simulink model "Linear_Test"  (R2025b)
settings: Solver=ode3  StartTime=0.0  StopTime=10.0  FixedStep=0.005  RelTol=1e-3
undefined symbols (not defined in the file or in its folder): SimPar
settings Model: Creator=bullo  LastModifiedBy=bullo

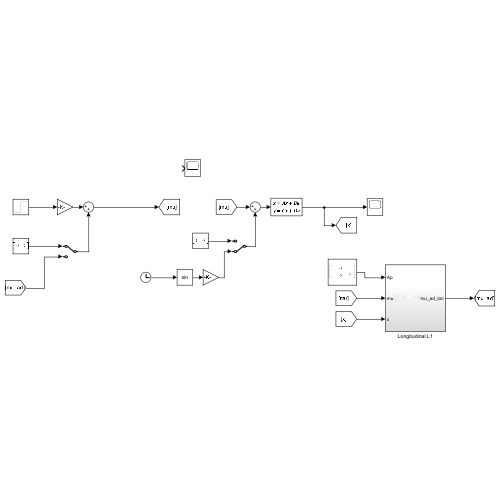
[thumbnail: Simulink's stored preview of the top-level diagram]
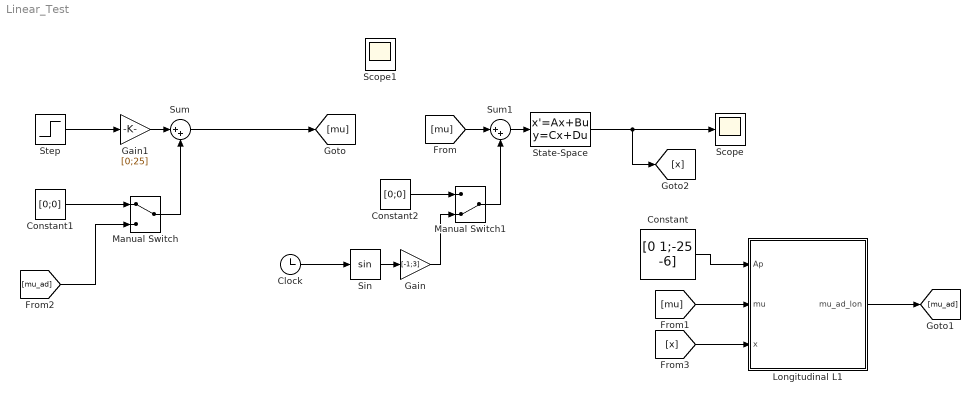
== system Linear_Test ==
  Clock : Clock
  Constant : Constant  Value=[0 1;-25 -6]
  Constant1 : Constant  Value=[0;0]
  Constant2 : Constant  Value=[0;0]
  Gain : Gain  Gain=[-1;3]
  Gain1 : Gain  Gain=[0;25]
  Longitudinal L1 : Subsystem
  Manual Switch : ManualSwitch
  Manual Switch1 : ManualSwitch  CurrentSetting=0
  Scope : Scope
      settings: ActiveDisplayYMinimum=-1.5712970754637268  ActiveDisplayYMaximum=3.9637552838320249
  Scope1 : Scope
      settings: ActiveDisplayYMinimum=-1  ActiveDisplayYMaximum=1
  Sin : Trigonometry
  State-Space : StateSpace  A=[0 1;-25 -6]  B=eye(2)  C=eye(2)  D=zeros(2,2)  InitialCondition=[0;0]
  Step : Step  SampleTime=0
  Sum : Sum  Inputs=|++
  Sum1 : Sum  Inputs=|++
  wires:
  State-Space/1 -> [x], Scope/1
  Constant/1 -> Longitudinal L1/1(Ap)
  [mu] -> Longitudinal L1/2(mu)
  Manual Switch/1 -> Sum/2
  [mu_ad] -> Manual Switch/2
  Longitudinal L1/1(mu_ad_lon) -> [mu_ad]
  [x] -> Longitudinal L1/3(x)
  [mu] -> Sum1/1
  Sum1/1 -> State-Space/1
  Manual Switch1/1 -> Sum1/2
  Constant2/1 -> Manual Switch1/1
  Clock/1 -> Sin/1
  Sin/1 -> Gain/1
  Gain/1 -> Manual Switch1/2
  Constant1/1 -> Manual Switch/1
  Step/1 -> Gain1/1
  Gain1/1 -> Sum/1
  Sum/1 -> [mu]

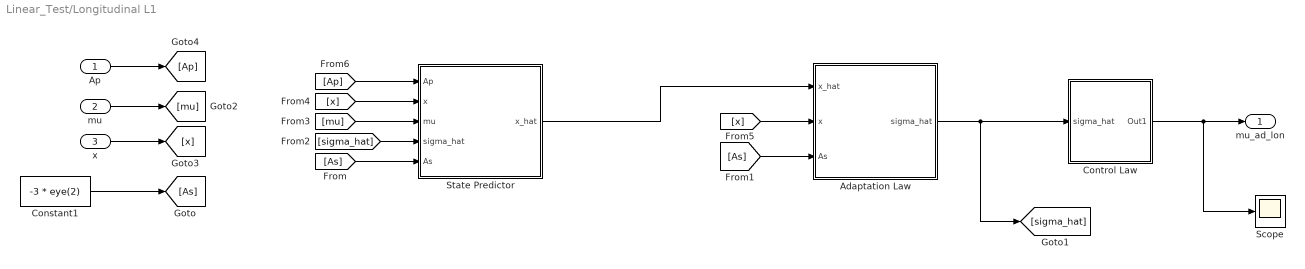
== system Linear_Test/Longitudinal L1 ==
  Ap : Inport
  mu : Inport  Port=2
  x : Inport  Port=3
  Adaptation Law : Subsystem
  Constant1 : Constant  Value=-3 * eye(2)
  Control Law : Subsystem
  Scope : Scope
      settings: ActiveDisplayYMinimum=-3.69393832537808  ActiveDisplayYMaximum=3.69393850364036  DataLoggingVariableName=ScopeData2
  State Predictor : Subsystem
  mu_ad_lon : Outport
  wires:
  Control Law/1(Out1) -> Scope/1, mu_ad_lon/1
  State Predictor/1(x_hat) -> Adaptation Law/1(x_hat)
  [As] -> Adaptation Law/3(As)
  Adaptation Law/1(sigma_hat) -> Control Law/1(sigma_hat), [sigma_hat]
  [sigma_hat] -> State Predictor/4(sigma_hat)
  [As] -> State Predictor/5(As)
  [mu] -> State Predictor/3(mu)
  [x] -> State Predictor/2(x)
  [x] -> Adaptation Law/2(x)
  [Ap] -> State Predictor/1(Ap)
  Constant1/1 -> [As]
  mu/1 -> [mu]
  Ap/1 -> [Ap]
  x/1 -> [x]

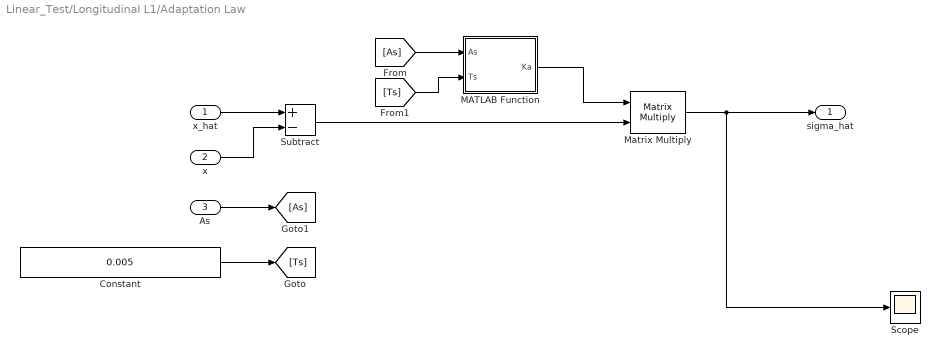
== system Linear_Test/Longitudinal L1/Adaptation Law ==
  x_hat : Inport
  x : Inport  Port=2
  As : Inport  Port=3
  Constant : Constant  Value=0.005
  MATLAB Function : MATLAB Function  TreatAsAtomicUnit=on
  Matrix Multiply : Product  Multiplication=Matrix(*)
  Scope : Scope
      settings: ActiveDisplayYMinimum=-49.625937496484333  ActiveDisplayYMaximum=446.63343746835915  DataLoggingVariableName=ScopeData14
  Subtract : Sum  Inputs=+-
  sigma_hat : Outport
  wires:
  x_hat/1 -> Subtract/1
  x/1 -> Subtract/2
  As/1 -> [As]
  [As] -> MATLAB Function/1(As)
  [Ts] -> MATLAB Function/2(Ts)
  MATLAB Function/1(Ka) -> Matrix Multiply/1
  Subtract/1 -> Matrix Multiply/2
  Constant/1 -> [Ts]
  Matrix Multiply/1 -> Scope/1, sigma_hat/1

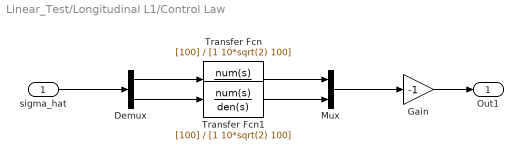
== system Linear_Test/Longitudinal L1/Control Law ==
  sigma_hat : Inport
  Demux : Demux  Outputs=2
  Gain : Gain  Gain=-1
  Mux : Mux  Inputs=2
  Transfer Fcn : TransferFcn  Numerator=[100]  Denominator=[1 10*sqrt(2) 100]
  Transfer Fcn1 : TransferFcn  Numerator=[100]  Denominator=[1 10*sqrt(2) 100]
  Out1 : Outport
  wires:
  Gain/1 -> Out1/1
  sigma_hat/1 -> Demux/1
  Demux/1 -> Transfer Fcn/1
  Transfer Fcn/1 -> Mux/1
  Demux/2 -> Transfer Fcn1/1
  Transfer Fcn1/1 -> Mux/2
  Mux/1 -> Gain/1

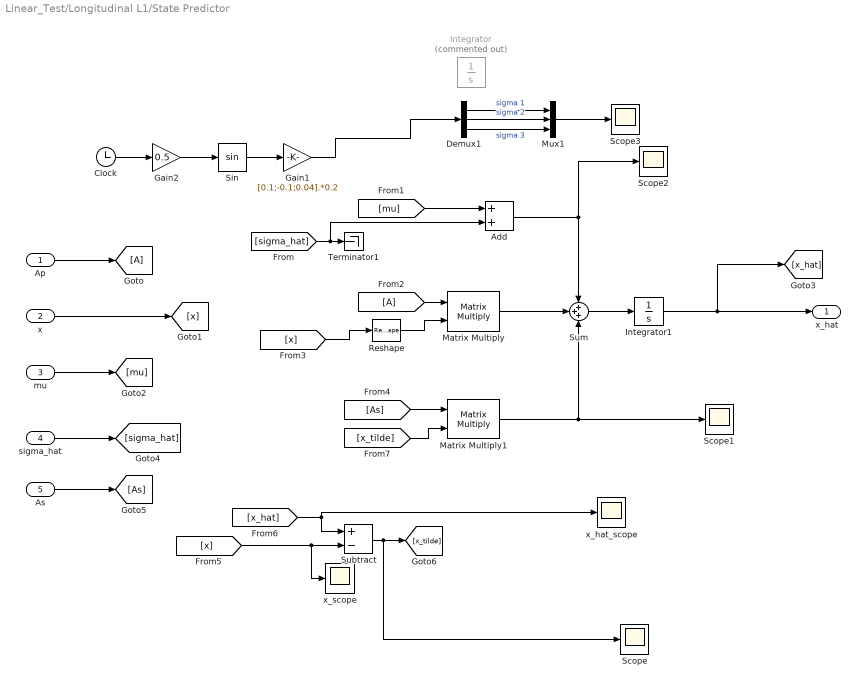
== system Linear_Test/Longitudinal L1/State Predictor ==
  Ap : Inport
  x : Inport  Port=2
  mu : Inport  Port=3
  sigma_hat : Inport  Port=4
  As : Inport  Port=5
  Add : Sum
  Clock : Clock
  Demux1 : Demux  Outputs=3
  From2 : From
  Gain1 : Gain  Gain=[0.1;-0.1;0.04].*0.2
  Gain2 : Gain  Gain=0.5
  Goto : Goto
  Integrator : Integrator  Commented=on  InitialCondition=[SimPar.EOM.Vel_bEb; SimPar.EOM.Omeg_BIb; SimPar.EOM.Pos_bii; SimPar.EOM.Q_i2b]  LimitOutput=on  UpperSaturationLimit=[inf; inf; inf; 10; 10; 10; inf; inf; inf; 1; 1; 1; 1]  LowerSaturationLimit=-[inf; inf; inf; 10; 10; 10; inf; inf; inf; 1; 1; 1; 1]  ContinuousStateAttributes='EOMStates'
  Integrator1 : Integrator  InitialCondition=zeros(2,1)
  Matrix Multiply : Product  Multiplication=Matrix(*)
  Matrix Multiply1 : Product  Multiplication=Matrix(*)
  Mux1 : Mux  Inputs=3
  Reshape : Reshape  OutputDimensionality=Column vector (2-D)
  Scope{,1..3} (4 alike) : Scope
      Scope settings: ActiveDisplayYMinimum=-2.2499999999999885  ActiveDisplayYMaximum=0.24999999999989467  DataLoggingVariableName=ScopeData7
      Scope1 settings: ActiveDisplayYMinimum=-1  ActiveDisplayYMaximum=1  DataLoggingVariableName=ScopeData10
      Scope2 settings: ActiveDisplayYMinimum=-42.220961000693308  ActiveDisplayYMaximum=273.95633453806431  DataLoggingVariableName=ScopeData13
      Scope3 settings: ActiveDisplayYMinimum=-0.024999999845933065  ActiveDisplayYMaximum=0.024999999845933065  DataLoggingVariableName=ScopeData15
  Sin : Trigonometry
  Subtract : Sum  Inputs=+-
  Sum : Sum  Inputs=+++
  Terminator1 : Terminator
  x_hat_scope : Scope
      settings: ActiveDisplayYMinimum=-0.7863916746849442  ActiveDisplayYMaximum=2.6267070904435581  DataLoggingVariableName=ScopeData8
  x_scope : Scope
      settings: ActiveDisplayYMinimum=-1  ActiveDisplayYMaximum=1  DataLoggingVariableName=ScopeData9
  x_hat : Outport
  wires:
  Demux1/2 -> Mux1/2  "sigma 2"
  Demux1/3 -> Mux1/3  "sigma 3"
  Gain1/1 -> Demux1/1
  Demux1/1 -> Mux1/1  "sigma 1"
  Mux1/1 -> Scope3/1
  Gain2/1 -> Sin/1
  [sigma_hat] -> Terminator1/1, Add/2
  Sin/1 -> Gain1/1
  Clock/1 -> Gain2/1
  Ap/1 -> Goto/1
  mu/1 -> [mu]
  Integrator1/1 -> x_hat/1, [x_hat]
  Sum/1 -> Integrator1/1
  Matrix Multiply/1 -> Sum/2
  From2/1 -> Matrix Multiply/1
  [x] -> Reshape/1
  [mu] -> Add/1
  Add/1 -> Scope2/1, Sum/1
  As/1 -> [As]
  Matrix Multiply1/1 -> Scope1/1, Sum/3
  [As] -> Matrix Multiply1/1
  [x] -> x_scope/1, Subtract/2
  [x_hat] -> x_hat_scope/1, Subtract/1
  Subtract/1 -> Scope/1, [x_tilde]
  [x_tilde] -> Matrix Multiply1/2
  Reshape/1 -> Matrix Multiply/2
  x/1 -> [x]
  sigma_hat/1 -> [sigma_hat]

== matlab function Linear_Test/Longitudinal L1/Adaptation Law/MATLAB Function ==
  data: As input; Ts input; Ka output
function Ka = fcn(As, Ts)

mat_exp = expm(As * Ts);
As_inv = pinv(As);

Ka = - pinv(As_inv * (mat_exp - eye(2))) * mat_exp;

end
